simulink model "A_3_5"  (R2023a)
settings: Solver=VariableStepAuto  StartTime=0.0  StopTime=10.0  RelTol=1e-3
settings Model: Creator=KEREM  LastModifiedBy=KEREM

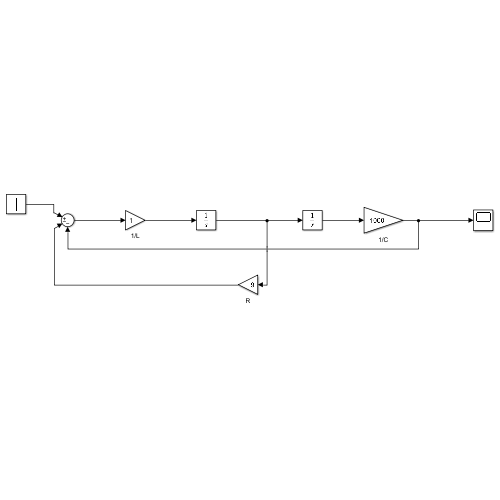
[thumbnail: Simulink's stored preview of the top-level diagram]
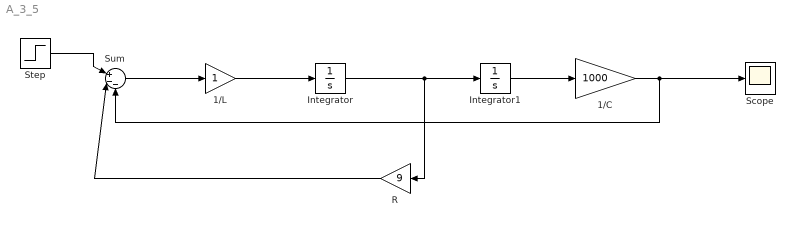
== system A_3_5 ==
  1/C : Gain  Gain=1000
  1/L : Gain
  Integrator : Integrator
  Integrator1 : Integrator
  R : Gain  Gain=9
  Scope : Scope
  Step : Step  SampleTime=0
  Sum : Sum  Inputs=|+--
  wires:
  Integrator1/1 -> 1/C/1
  Sum/1 -> 1/L/1
  1/L/1 -> Integrator/1
  Integrator/1 -> R/1, Integrator1/1
  R/1 -> Sum/2
  1/C/1 -> Scope/1, Sum/3
  Step/1 -> Sum/1
